simulink model "PCCi_DCM"  (R2022b)
settings: Solver=FixedStepDiscrete  StartTime=0.0  StopTime=1  FixedStep=0.001  RelTol=1e-3
settings Model: Creator=realj  LastModifiedBy=realj
settings OptimizationCC: DefaultParameterBehavior=Inlined  EnhancedBackFolding=on  PassReuseOutputArgsAs=Individual arguments  ZeroExternalMemoryAtStartup=off  ZeroInternalMemoryAtStartup=off  OptimizeBlockOrder=speed  DifferentSizesBufferReuse=on  OptimizationCustomize=off  EfficientTunableParamExpr=on
settings DebuggingCC: ParameterTunabilityLossMsg=error
settings SFSimCC: MATLABDynamicMemAlloc=off
settings RTWCC: Description=Embedded Coder  SystemTargetFile=ert.tlc  GenCodeOnly=on  TemplateMakefile=ert_default_tmf  GenerateReport=on  LaunchReport=on
settings CodeAppCC: ForceParamTrailComments=on  IgnoreCustomStorageClasses=off  OperatorAnnotations=on  SimulinkDataObjDesc=on  SFDataObjDesc=on  InsertBlockDesc=on
settings ERTTargetCC: TargetLangStandard=C99 (ISO)  GenerateSampleERTMain=on  InlinedParameterPlacement=NonHierarchical  ERTCustomFileTemplate=example_file_process.tlc

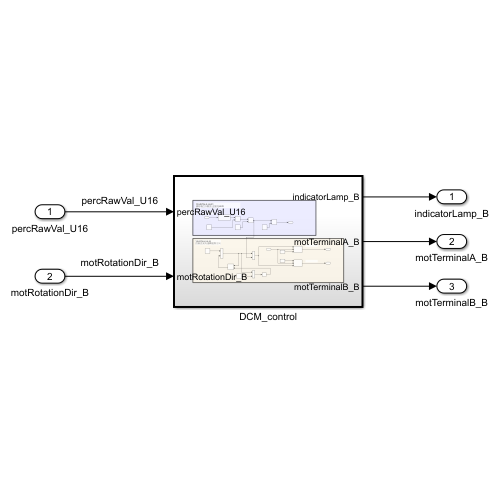
[thumbnail: Simulink's stored preview of the top-level diagram]
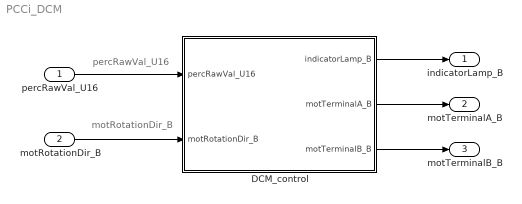
== system PCCi_DCM ==
  note: motRotationDir_B
  note: percRawVal_U16
  percRawVal_U16 : Inport  OutDataTypeStr=uint16
  motRotationDir_B : Inport  Port=2  OutDataTypeStr=boolean
  DCM_control : Subsystem  TreatAsAtomicUnit=on
      settings: RTWFcnNameOpts=Use subsystem name  RTWFileNameOpts=Use subsystem name
  indicatorLamp_B : Outport
  motTerminalA_B : Outport  Port=2  OutDataTypeStr=boolean
  motTerminalB_B : Outport  Port=3  OutDataTypeStr=boolean
  wires:
  percRawVal_U16/1 -> DCM_control/1(percRawVal_U16)
  DCM_control/1(indicatorLamp_B) -> indicatorLamp_B/1
  DCM_control/2(motTerminalA_B) -> motTerminalA_B/1
  DCM_control/3(motTerminalB_B) -> motTerminalB_B/1
  motRotationDir_B/1 -> DCM_control/2(motRotationDir_B)

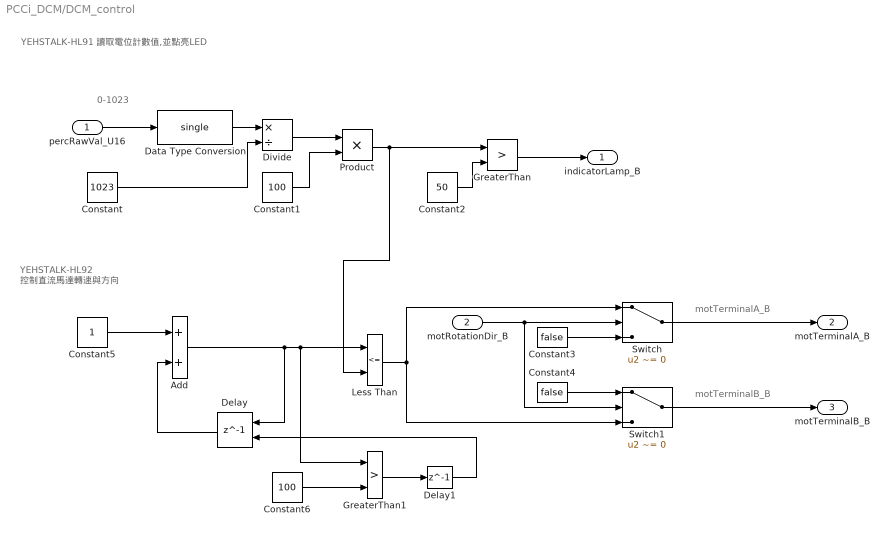
== system PCCi_DCM/DCM_control ==
  note: YEHSTALK-HL92
      | 控制直流馬達轉速與方向
  note: YEHSTALK-HL91
      | 讀取電位計數值,並點亮LED
  note: motTerminalB_B
  note: motTerminalA_B
  note: 0-1023
  percRawVal_U16 : Inport  OutDataTypeStr=uint16
  motRotationDir_B : Inport  Port=2  OutDataTypeStr=boolean
  Add : Sum
  Constant : Constant  Value=1023  OutDataTypeStr=single
  Constant1 : Constant  Value=100  OutDataTypeStr=int8
  Constant2 : Constant  Value=50  OutDataTypeStr=int8
  Constant3 : Constant  Value=false  OutDataTypeStr=boolean
  Constant4 : Constant  Value=false  OutDataTypeStr=boolean
  Constant5 : Constant  OutDataTypeStr=int8
  Constant6 : Constant  Value=100  OutDataTypeStr=int8
  Data Type Conversion : DataTypeConversion  OutDataTypeStr=single  SaturateOnIntegerOverflow=off  RndMeth=Floor
  Delay : Delay  DelayLength=1  ExternalReset=Rising
      settings: InputPortMap=u0,r5
  Delay1 : Delay  DelayLength=1
  Divide : Product  Inputs=*/
  GreaterThan : RelationalOperator  Operator=>  OutDataTypeStr=boolean  RndMeth=Simplest  InputSameDT=off
  GreaterThan1 : RelationalOperator  Operator=>  OutDataTypeStr=boolean  RndMeth=Simplest  InputSameDT=off
  Less Than : RelationalOperator  Operator=<=  OutDataTypeStr=boolean  RndMeth=Simplest  InputSameDT=off
  Product : Product
  Switch : Switch  Criteria=u2 ~= 0  SaturateOnIntegerOverflow=off  InputSameDT=off
  Switch1 : Switch  Criteria=u2 ~= 0  SaturateOnIntegerOverflow=off  InputSameDT=off
  indicatorLamp_B : Outport
  motTerminalA_B : Outport  Port=2  OutDataTypeStr=boolean
  motTerminalB_B : Outport  Port=3  OutDataTypeStr=boolean
  wires:
  percRawVal_U16/1 -> Data Type Conversion/1
  Data Type Conversion/1 -> Divide/1
  Constant/1 -> Divide/2
  Constant1/1 -> Product/2
  Product/1 -> Less Than/2, GreaterThan/1
  Constant2/1 -> GreaterThan/2
  GreaterThan/1 -> indicatorLamp_B/1
  Switch/1 -> motTerminalA_B/1
  Switch1/1 -> motTerminalB_B/1
  motRotationDir_B/1 -> Switch/2, Switch1/2
  Constant3/1 -> Switch/3
  Constant4/1 -> Switch1/1
  Constant5/1 -> Add/1
  Add/1 -> GreaterThan1/1, Less Than/1, Delay/1
  Delay/1 -> Add/2
  Less Than/1 -> Switch/1, Switch1/3
  Constant6/1 -> GreaterThan1/2
  GreaterThan1/1 -> Delay1/1
  Delay1/1 -> Delay/2
  Divide/1 -> Product/1
